simulink model "const_vel_static_obst"  (R2023b)
settings: Solver=ode4  StartTime=0.0  StopTime=50  FixedStep=1e-3  RelTol=1e-3  EnableMultiTasking=on
values from neighbouring files (symbols this model uses):
  Ts = 0.01    [const_vel_static_obst_run.m]    (also in const_vel_wall_run.m; run_acceleration.m; run_template.m; simple_const_vel_run.m)
  V_ref = 50/3.6    (= 13.8888888889)    [const_vel_static_obst_run.m]    (also in const_vel_wall_run.m; run_acceleration.m = 27.7777777778; run_template.m = 27.7777777778; simple_const_vel_run.m)
  X0 = [V_ref 0 0 0 0 0 0]    [const_vel_static_obst_run.m]    (also in const_vel_wall_run.m; run_acceleration.m = [V_ref 0 0 0 0 0]; run_template.m; simple_const_vel_run.m)
undefined symbols (not defined in the file or in its folder): data, init, input
settings Model: Creator=bshyrokau  LastModifiedBy=maart
settings SolverCC: AlgebraicLoopSolver=TrustRegion  AutoInsertRateTranBlk=on
settings DataIOCC: SaveOutput=off  SignalLogging=off  DSMLogging=off  SaveTime=off  ReturnWorkspaceOutputs=off
settings OptimizationCC: ReuseModelBlockBuffer=off  LifeSpan=inf
settings DebuggingCC: UnconnectedInputMsg=warning  UnconnectedOutputMsg=warning  UnconnectedLineMsg=warning  AllowSymbolicDim=off  SFUnexpectedBacktrackingDiag=warning  SFNoUnconditionalDefaultTransitionDiag=warning  SFExecutionAtInitializationDiag=none  ArithmeticOperatorsInVariantConditions=warning
settings ModelReferenceCC: EnableRefExpFcnMdlSchedulingChecks=on  PropagateSignalLabelsOutOfModel=off
settings SFSimCC: SimUseLocalCustomCode=off  CustomCodeUndefinedFunction=UseInterfaceOnly
settings RTWCC: RTWUseLocalCustomCode=off
settings CodeAppCC: StateflowObjectComments=on
settings GRTTargetCC: TargetLangStandard=C89/C90 (ANSI)
settings ConfigComp: CovMetricSettings=dw  CovSaveCumulativeToWorkspaceVar=on  CovSaveSingleToWorkspaceVar=on  CovExternalEMLEnable=off
settings SimscapeCC: SimscapeNormalizeSystem=off
settings ConfigurationSet: Description=SimMechanics 2G

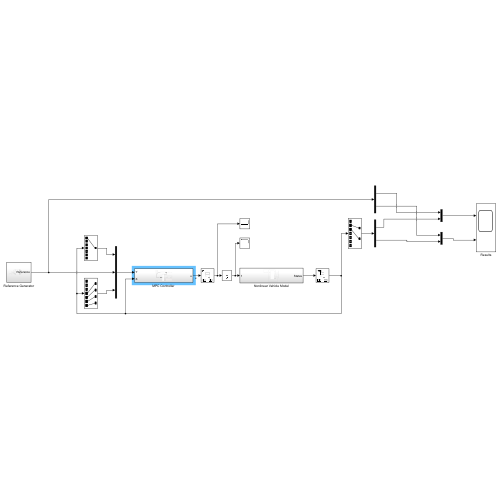
[thumbnail: Simulink's stored preview of the top-level diagram]
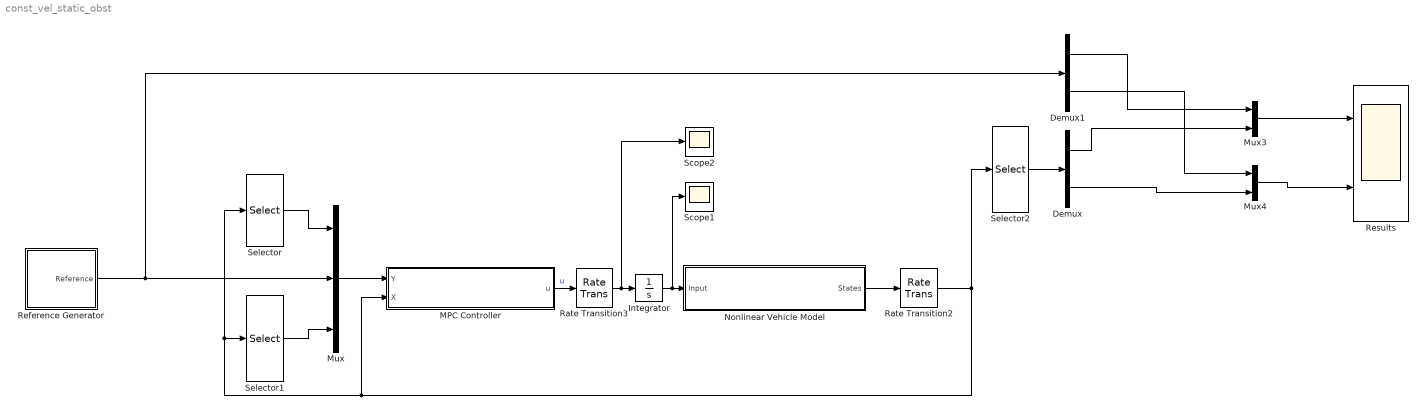
== system const_vel_static_obst ==
  Demux : Demux  Outputs=2
  Demux1 : Demux  Outputs=2
  Integrator : Integrator
  "MPC Controller " : Subsystem
  Mux : Mux  Inputs=3
  Mux3 : Mux  Inputs=2
  Mux4 : Mux  Inputs=2
  Nonlinear Vehicle Model : Subsystem
  Rate Transition2 : RateTransition  InitialCondition=X0  OutPortSampleTime=Ts
  Rate Transition3 : RateTransition  InitialCondition=[0]
  Reference Generator : Subsystem
  Results : Scope  NumInputPorts=2
  Scope1 : Scope
  Scope2 : Scope
  Selector : Selector  InputPortWidth=7  IndexOptions=Index vector (dialog)  Indices=[1]  OutputSizes=1
  Selector1 : Selector  InputPortWidth=7  IndexOptions=Index vector (dialog)  Indices=[4,5,6,7]  OutputSizes=1
  Selector2 : Selector  InputPortWidth=7  IndexOptions=Index vector (dialog)  Indices=[2,3]  OutputSizes=1
  wires:
  Nonlinear Vehicle Model/1(States) -> Rate Transition2/1
  Rate Transition2/1 -> "MPC Controller "/2(X), Selector/1, Selector1/1, Selector2/1
  "MPC Controller "/1(u) -> Rate Transition3/1  "u"
  Mux/1 -> "MPC Controller "/1(Y)
  Selector1/1 -> Mux/3
  Selector2/1 -> Demux/1
  Demux1/1 -> Mux3/1
  Demux1/2 -> Mux4/1
  Demux/1 -> Mux3/2
  Demux/2 -> Mux4/2
  Reference Generator/1(Reference) -> Demux1/1, Mux/2
  Selector/1 -> Mux/1
  Rate Transition3/1 -> Scope2/1, Integrator/1
  Integrator/1 -> Scope1/1, Nonlinear Vehicle Model/1(Input)
  Mux3/1 -> Results/1
  Mux4/1 -> Results/2

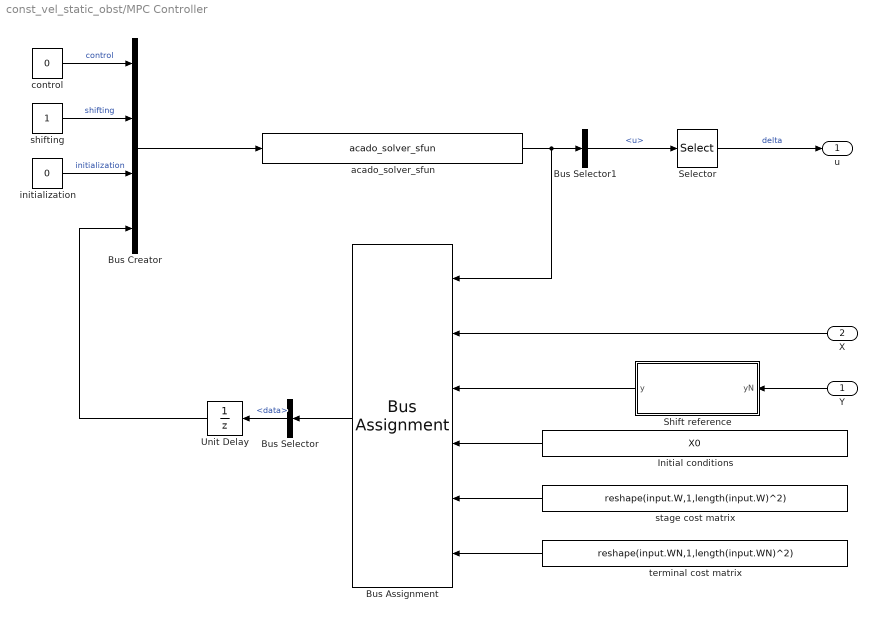
== system const_vel_static_obst/MPC Controller  ==
  Y : Inport
  X : Inport  Port=2
  Bus Assignment : BusAssignment  AssignedSignals=data.x0,data.y,data.yN,data.W,data.WN
  Bus Creator : BusCreator  Inputs=4  OutDataTypeStr=Bus: ACADOinput
  Bus Selector : BusSelector  OutputSignals=data
  Bus Selector1 : BusSelector  OutputSignals=data.u
  Initial conditions : Constant  Value=X0
  Selector : Selector  InputPortWidth=Np  IndexOptions=Starting index (dialog)  Indices=1  OutputSizes=1
  Shift reference : MATLAB Function  TreatAsAtomicUnit=on
  Unit Delay : UnitDelay  InitialCondition=init  SampleTime=Ts  HasFrameUpgradeWarning=on
  acado_solver_sfun : S-Function  FunctionName=acado_solver_sfun  SFunctionDeploymentMode=off  EnableBusSupport=off  mask(Legacy Function){SFunctionSpec=acado_step(ACADOinput u1[1], ACADOoutput y1[1]), ShowSpec=on}
      mask prompts: ShowSpec "Display function specification"
      mask help:
      | This block allows you to call the legacy functions specified by the following Legacy Code Tool definition:
      | def.SFunctionName = 'acado_solver_sfun';
      | def.OutputFcnSpec = 'acado_step(ACADOinput u1[1], ACADOoutput y1[1])';
      | def.StartFcnSpec = 'acado_initialize( void )';
      | def.TerminateFcnSpec = 'acado_cleanup( void )';
      | def.HeaderFiles = {'acado_common.h', 'acado_solver_sfunction.h'};
      | def.SourceFiles = {'acado_solver.c', 'acado_integrator.c', 'acado_auxiliary_functions.c', 'acado_solver_sfunction.c', 'acado_qpoases3_interface.c', 'qpoases3\src\Bounds.c', 'qpoases3\src\Constraints.c', 'qpoases3\src\Indexlist.c', 'qpoases3\src\Matrices.c', 'qpoases3\src\MessageHandling.c', 'qpoases3\src\Options.c', 'qpoases3\src\Flipper.c', 'qpoases3\src\QProblem.c', 'qpoases3\src\QProblemB.c', 'qpoases3\src\Utils.c'};
      mask Help: <p>This block was generated automatically by the Legacy Code Tool. For detailed help on this tool, call<a href="matlab:legacy_code('help')"> legacy_code('help')</a>.</p>
      mask Callback ShowSpec:
      | if strcmp(get_param(gcbh, 'ShowSpec'), 'on')
      |   set_param(gcbh, 'MaskDisplay', sprintf('fprintf(''%s'');', get_param(gcbh, 'SFunctionSpec')));
      | else
      |   set_param(gcbh, 'MaskDisplay', sprintf('fprintf(''%s'');', get_param(gcbh, 'FunctionName')));
      | end
      mask Display: fprintf('acado_step(ACADOinput u1[1], ACADOoutput y1[1])');
  control : Constant  Value=0  OutDataTypeStr=int32
  initialization : Constant  Value=0  OutDataTypeStr=int32
  shifting : Constant  OutDataTypeStr=int32
  stage cost matrix : Constant  Value=reshape(input.W,1,length(input.W)^2)
  terminal cost matrix : Constant  Value=reshape(input.WN,1,length(input.WN)^2)
  u : Outport
  wires:
  control/1 -> Bus Creator/1  "control"
  Bus Selector1/1 -> Selector/1  "<u>"
  initialization/1 -> Bus Creator/3  "initialization"
  acado_solver_sfun/1 -> Bus Selector1/1, Bus Assignment/1
  shifting/1 -> Bus Creator/2  "shifting"
  X/1 -> Bus Assignment/2
  Bus Assignment/1 -> Bus Selector/1
  terminal cost matrix/1 -> Bus Assignment/6
  Initial conditions/1 -> Bus Assignment/4
  Shift reference/1(y) -> Bus Assignment/3
  stage cost matrix/1 -> Bus Assignment/5
  Bus Selector/1 -> Unit Delay/1  "<data>"
  Unit Delay/1 -> Bus Creator/4
  Bus Creator/1 -> acado_solver_sfun/1
  Selector/1 -> u/1  "delta"
  Y/1 -> Shift reference/1(yN)

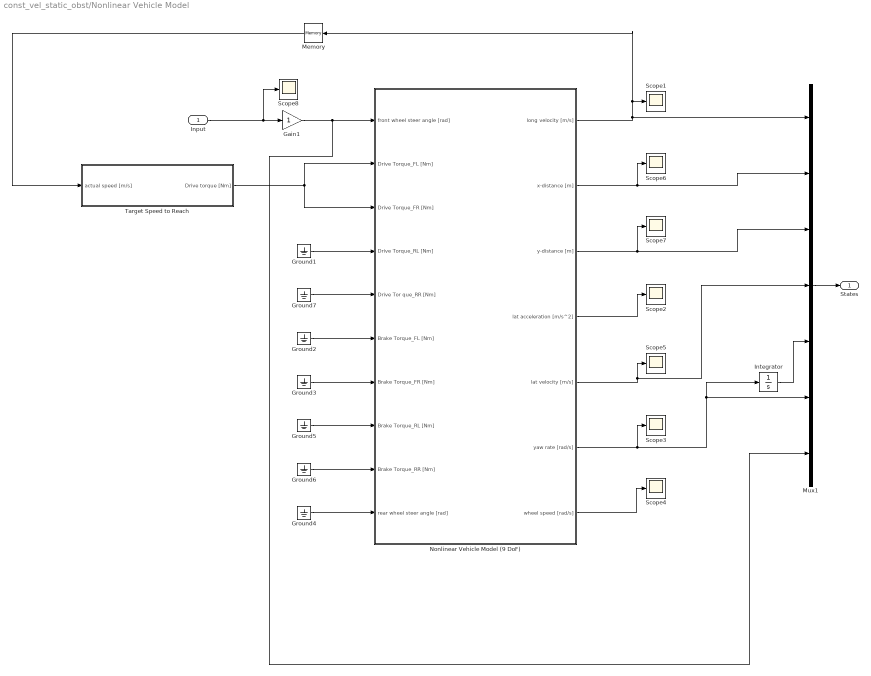
== system const_vel_static_obst/Nonlinear Vehicle Model ==
  Input : Inport
  Gain1 : Gain
  Ground{1..7} (7 alike) : Ground
  Integrator : Integrator
  Memory : Memory
  Mux1 : Mux  Inputs=7
  Nonlinear Vehicle Model (9 DoF) : Subsystem
      mask help: Simulink:masks:GenSFuncDesc_MD
      mask Help: eval('feval(''rtwprivate'',''rtwhelpview'',''rtw_sfcn_block'')');
  Scope{1..8} (8 alike) : Scope
  Target Speed to Reach : Subsystem
  States : Outport
  wires:
  Nonlinear Vehicle Model (9 DoF)/2(x-distance [m]) -> Mux1/2, Scope6/1
  Input/1 -> Scope8/1, Gain1/1
  Nonlinear Vehicle Model (9 DoF)/5(lat velocity [m/s]) -> Scope5/1, Mux1/4
  Ground3/1 -> Nonlinear Vehicle Model (9 DoF)/7(Brake Torque_FR [Nm])
  Nonlinear Vehicle Model (9 DoF)/3(y-distance [m]) -> Mux1/3, Scope7/1
  Nonlinear Vehicle Model (9 DoF)/1(long velocity [m/s]) -> Memory/1, Scope1/1, Mux1/1
  Nonlinear Vehicle Model (9 DoF)/4(lat acceleration [m/s^2]) -> Scope2/1
  Nonlinear Vehicle Model (9 DoF)/6(yaw rate [rad/s]) -> Scope3/1, Mux1/6, Integrator/1
  Ground2/1 -> Nonlinear Vehicle Model (9 DoF)/6(Brake Torque_FL [Nm])
  Mux1/1 -> States/1
  Integrator/1 -> Mux1/5
  Ground4/1 -> Nonlinear Vehicle Model (9 DoF)/10(rear wheel steer angle [rad])
  Ground5/1 -> Nonlinear Vehicle Model (9 DoF)/8(Brake Torque_RL [Nm])
  Ground6/1 -> Nonlinear Vehicle Model (9 DoF)/9(Brake Torque_RR [Nm])
  Nonlinear Vehicle Model (9 DoF)/7(wheel speed [rad/s]) -> Scope4/1
  Target Speed to Reach/1(Drive torque [Nm]) -> Nonlinear Vehicle Model (9 DoF)/3(Drive Torque_FR [Nm]), Nonlinear Vehicle Model (9 DoF)/2(Drive Torque_FL [Nm])
  Gain1/1 -> Nonlinear Vehicle Model (9 DoF)/1(front wheel steer angle [rad]), Mux1/7
  Ground7/1 -> Nonlinear Vehicle Model (9 DoF)/5(Drive Tor	que_RR [Nm])
  Ground1/1 -> Nonlinear Vehicle Model (9 DoF)/4(Drive Torque_RL [Nm])
  Memory/1 -> Target Speed to Reach/1(actual speed [m/s])

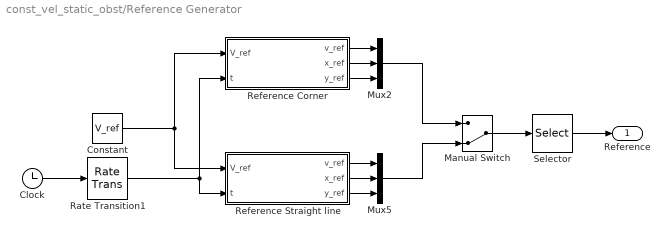
== system const_vel_static_obst/Reference Generator ==
  Clock : Clock
  Constant : Constant  Value=V_ref
  Manual Switch : ManualSwitch  CurrentSetting=0
  Mux2 : Mux  Inputs=3
  Mux5 : Mux  Inputs=3
  Rate Transition1 : RateTransition  OutPortSampleTime=Ts
  Reference Corner : MATLAB Function  TreatAsAtomicUnit=on
  Reference Straight line : MATLAB Function  TreatAsAtomicUnit=on
  Selector : Selector  InputPortWidth=3  IndexOptions=Index vector (dialog)  Indices=[2 3]  OutputSizes=1
  Reference : Outport
  wires:
  Clock/1 -> Rate Transition1/1
  Reference Corner/2(x_ref) -> Mux2/2
  Reference Corner/1(v_ref) -> Mux2/1
  Rate Transition1/1 -> Reference Straight line/2(t), Reference Corner/2(t)
  Constant/1 -> Reference Straight line/1(V_ref), Reference Corner/1(V_ref)
  Reference Corner/3(y_ref) -> Mux2/3
  Reference Straight line/1(v_ref) -> Mux5/1
  Reference Straight line/2(x_ref) -> Mux5/2
  Reference Straight line/3(y_ref) -> Mux5/3
  Selector/1 -> Reference/1
  Mux5/1 -> Manual Switch/2
  Mux2/1 -> Manual Switch/1
  Manual Switch/1 -> Selector/1

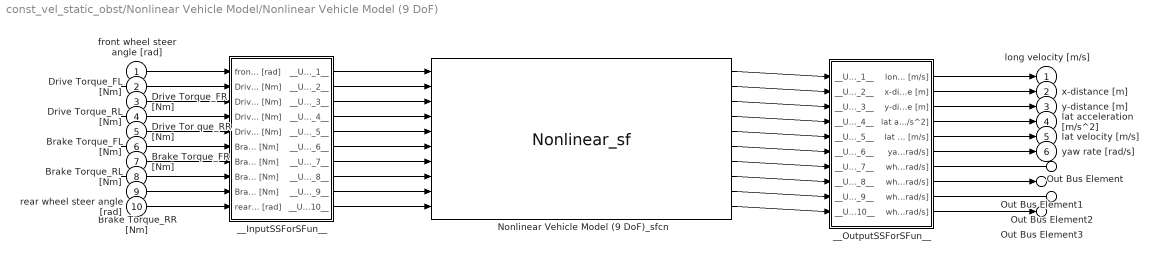
== system const_vel_static_obst/Nonlinear Vehicle Model/Nonlinear Vehicle Model (9 DoF) ==
  front wheel steer angle [rad] : Inport
  Drive Torque_FL [Nm] : Inport  Port=2
  Drive Torque_FR [Nm] : Inport  Port=3
  Drive Torque_RL [Nm] : Inport  Port=4
  Drive Tor	que_RR [Nm] : Inport  Port=5
  Brake Torque_FL [Nm] : Inport  Port=6
  Brake Torque_FR [Nm] : Inport  Port=7
  Brake Torque_RL [Nm] : Inport  Port=8
  Brake Torque_RR [Nm] : Inport  Port=9
  rear wheel steer angle [rad] : Inport  Port=10
  Nonlinear Vehicle Model (9 DoF)_sfcn : S-Function  FunctionName=Nonlinear_sf  SFunctionModules=""  SFunctionDeploymentMode=off  EnableBusSupport=off  mask{rtw_sf_name=Nonlinear_sf, showVar=off}
      mask prompts: rtw_sf_name "Simulink:masks:GenSFuncName_MP"; showVar "Simulink:masks:GenSFuncShowModuleList_MP"
      mask help: Simulink:masks:GenSFuncDesc_MD
      mask init:
      | displist = '';
      | if ~strcmp(get_param(gcb, 'FunctionName'), rtw_sf_name);
      |   set_param(gcb, 'FunctionName', rtw_sf_name);
      | end
      | % Check if we are generating code
      | rtw_mode = false;
      | if strcmpi(get_param(bdroot(gcb),'SimulationStatus'),'Initializing')
      | 	rtw_mode = strcmpi(get_param(bdroot(gcb),'BuildingRTWCode'),'on') && ...
      | 		~strcmpi(get_param(bdroot(gcb),'TargetStyle'),'SimulationTarget');
      | end
      | if showVar || rtw_mode
      | 	if exist('rtwsfunc') == 2 | exist('rtwsfunc') == 6
      | 		tmplist = rtwsfunc(rtw_sf_name,gcb);
      | 		tmplist = DAStudio.message('Simulink:masks:GenSFuncListOfModules_IC', tmplist);
      | 	elseif showVar
      | 		tmplist1 = DAStudio.message('Simulink:masks:GenSFuncListOfModules_IC', '');
      |         tmplist2 = DAStudio.message('Simulink:masks:GenSFuncNotLicensed_IC');
      |         tmplist = [tmplist1 tmplist2];
      |  	end
      | end
      | if showVar
      |   displist = tmplist;
      | end
      settings: CopyFcn=|
      | if ~strcmp(get_param(gcb,'Linkstatus'),'none') && ...
      | ~strcmp(get_param(gcb,'Linkstatus'),'implicit')
      |   set_param(gcb,'LinkStatus','none');
      | end
      mask Help: eval('feval(''rtwprivate'',''rtwhelpview'',''rtw_sfcn_block'')');
      mask Display:
      | port_label('input',1,'front wheel steer angle [rad]');
      | port_label('input',2,'Drive Torque_FL [Nm]');
      | port_label('input',3,'Drive Torque_FR [Nm]');
      | port_label('input',4,'Drive Torque_RL [Nm]');
      | port_label('input',5,'Drive Tor	que_RR [Nm]');
      | port_label('input',6,'Brake Torque_FL [Nm]');
      | port_label('input',7,'Brake Torque_FR [Nm]');
      | port_label('input',8,'Brake Torque_RL [Nm]');
      | port_label('input',9,'Brake Torque_RR [Nm]');
      | port_label('input',10,'rear wheel steer angle [rad]');
      | port_label('output',1,'long velocity [m/s]');
      | port_label('output',2,'x-distance [m]');
      | port_label('output',3,'y-distance [m]');
      | port_label('output',4,'lat acceleration [m/s^2]');
      | port_label('output',5,'lat velocity [m/s]');
      | port_label('output',6,'yaw rate [rad/s]');
      | port_label('output',7,'wheel speed FL [rad/s]');
      | port_label('output',8,'wheel speed FR [rad/s]');
      | port_label('output',9,'wheel speed RL [rad/s]');
      | port_label('output',10,'wheel speed RR [rad/s]');
  __InputSSForSFun__ : Subsystem
  __OutputSSForSFun__ : Subsystem
  long velocity [m/s] : Outport  VectorParamsAs1DForOutWhenUnconnected=off
  x-distance [m] : Outport  Port=2  VectorParamsAs1DForOutWhenUnconnected=off
  y-distance [m] : Outport  Port=3  VectorParamsAs1DForOutWhenUnconnected=off
  lat acceleration [m/s^2] : Outport  Port=4  VectorParamsAs1DForOutWhenUnconnected=off
  lat velocity [m/s] : Outport  Port=5  VectorParamsAs1DForOutWhenUnconnected=off
  yaw rate [rad/s] : Outport  Port=6  VectorParamsAs1DForOutWhenUnconnected=off
  Out Bus Element : Outport  Port=7  PortName=wheel speed [rad/s]  Element=wheel speed FL [rad/s]
  Out Bus Element1 : Outport  Port=7  PortName=wheel speed [rad/s]  Element=wheel speed FR [rad/s]
  Out Bus Element2 : Outport  Port=7  PortName=wheel speed [rad/s]  Element=wheel speed RL [rad/s]
  Out Bus Element3 : Outport  Port=7  PortName=wheel speed [rad/s]  Element=wheel speed RR [rad/s]
  wires:
  front wheel steer angle [rad]/1 -> __InputSSForSFun__/1(front wheel steer angle [rad])
  Drive Torque_FL [Nm]/1 -> __InputSSForSFun__/2(Drive Torque_FL [Nm])
  Drive Torque_FR [Nm]/1 -> __InputSSForSFun__/3(Drive Torque_FR [Nm])
  Drive Torque_RL [Nm]/1 -> __InputSSForSFun__/4(Drive Torque_RL [Nm])
  Drive Tor	que_RR [Nm]/1 -> __InputSSForSFun__/5(Drive Tor	que_RR [Nm])
  Brake Torque_FL [Nm]/1 -> __InputSSForSFun__/6(Brake Torque_FL [Nm])
  Brake Torque_FR [Nm]/1 -> __InputSSForSFun__/7(Brake Torque_FR [Nm])
  Brake Torque_RL [Nm]/1 -> __InputSSForSFun__/8(Brake Torque_RL [Nm])
  Brake Torque_RR [Nm]/1 -> __InputSSForSFun__/9(Brake Torque_RR [Nm])
  rear wheel steer angle [rad]/1 -> __InputSSForSFun__/10(rear wheel steer angle [rad])
  __InputSSForSFun__/1(__UniqueOutportName__1__) -> Nonlinear Vehicle Model (9 DoF)_sfcn/1
  __InputSSForSFun__/2(__UniqueOutportName__2__) -> Nonlinear Vehicle Model (9 DoF)_sfcn/2
  __InputSSForSFun__/3(__UniqueOutportName__3__) -> Nonlinear Vehicle Model (9 DoF)_sfcn/3
  __InputSSForSFun__/4(__UniqueOutportName__4__) -> Nonlinear Vehicle Model (9 DoF)_sfcn/4
  __InputSSForSFun__/5(__UniqueOutportName__5__) -> Nonlinear Vehicle Model (9 DoF)_sfcn/5
  __InputSSForSFun__/6(__UniqueOutportName__6__) -> Nonlinear Vehicle Model (9 DoF)_sfcn/6
  __InputSSForSFun__/7(__UniqueOutportName__7__) -> Nonlinear Vehicle Model (9 DoF)_sfcn/7
  __InputSSForSFun__/8(__UniqueOutportName__8__) -> Nonlinear Vehicle Model (9 DoF)_sfcn/8
  __InputSSForSFun__/9(__UniqueOutportName__9__) -> Nonlinear Vehicle Model (9 DoF)_sfcn/9
  __InputSSForSFun__/10(__UniqueOutportName__10__) -> Nonlinear Vehicle Model (9 DoF)_sfcn/10
  Nonlinear Vehicle Model (9 DoF)_sfcn/1 -> __OutputSSForSFun__/1(__UniqueInportName__1__)
  Nonlinear Vehicle Model (9 DoF)_sfcn/2 -> __OutputSSForSFun__/2(__UniqueInportName__2__)
  Nonlinear Vehicle Model (9 DoF)_sfcn/3 -> __OutputSSForSFun__/3(__UniqueInportName__3__)
  Nonlinear Vehicle Model (9 DoF)_sfcn/4 -> __OutputSSForSFun__/4(__UniqueInportName__4__)
  Nonlinear Vehicle Model (9 DoF)_sfcn/5 -> __OutputSSForSFun__/5(__UniqueInportName__5__)
  Nonlinear Vehicle Model (9 DoF)_sfcn/6 -> __OutputSSForSFun__/6(__UniqueInportName__6__)
  Nonlinear Vehicle Model (9 DoF)_sfcn/7 -> __OutputSSForSFun__/7(__UniqueInportName__7__)
  Nonlinear Vehicle Model (9 DoF)_sfcn/8 -> __OutputSSForSFun__/8(__UniqueInportName__8__)
  Nonlinear Vehicle Model (9 DoF)_sfcn/9 -> __OutputSSForSFun__/9(__UniqueInportName__9__)
  Nonlinear Vehicle Model (9 DoF)_sfcn/10 -> __OutputSSForSFun__/10(__UniqueInportName__10__)
  __OutputSSForSFun__/1(long velocity [m/s]) -> long velocity [m/s]/1
  __OutputSSForSFun__/2(x-distance [m]) -> x-distance [m]/1
  __OutputSSForSFun__/3(y-distance [m]) -> y-distance [m]/1
  __OutputSSForSFun__/4(lat acceleration [m/s^2]) -> lat acceleration [m/s^2]/1
  __OutputSSForSFun__/5(lat velocity [m/s]) -> lat velocity [m/s]/1
  __OutputSSForSFun__/6(yaw rate [rad/s]) -> yaw rate [rad/s]/1
  __OutputSSForSFun__/7(wheel speed FL [rad/s]) -> Out Bus Element/1
  __OutputSSForSFun__/8(wheel speed FR [rad/s]) -> Out Bus Element1/1
  __OutputSSForSFun__/9(wheel speed RL [rad/s]) -> Out Bus Element2/1
  __OutputSSForSFun__/10(wheel speed RR [rad/s]) -> Out Bus Element3/1

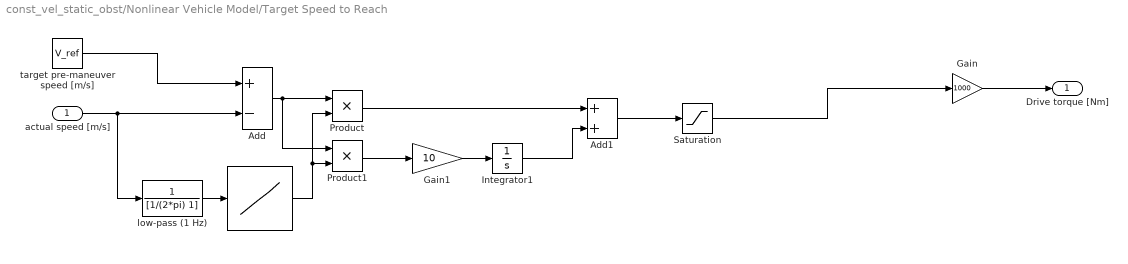
== system const_vel_static_obst/Nonlinear Vehicle Model/Target Speed to Reach ==
  actual speed [m/s] : Inport
  " " : Lookup_n-D  NumberOfTableDimensions=1  BreakpointsForDimension1="[-10  0  10 30]"  IndexSearchMethod=Linear search  Table=[0.1 0.1 1 1]  ExtrapMethod=Clip  RemoveProtectionInput=on  UseLastTableValue=on  RndMeth=Simplest
  Add : Sum  Inputs=+-
  Add1 : Sum
  Gain : Gain  Gain=1000
  Gain1 : Gain  Gain=10
  Integrator1 : Integrator  LimitOutput=on  UpperSaturationLimit=0.1  LowerSaturationLimit=-0.1
  Product : Product  RndMeth=Zero
  Product1 : Product  RndMeth=Zero
  Saturation : Saturate  UpperLimit=1  LowerLimit=0
  low-pass (1 Hz) : TransferFcn  Denominator=[1/(2*pi) 1]
  "target pre-maneuver speed [m/s] " : Constant  Value=V_ref
  Drive torque [Nm] : Outport
  wires:
  actual speed [m/s]/1 -> low-pass (1 Hz)/1, Add/2
  "target pre-maneuver speed [m/s] "/1 -> Add/1
  Gain1/1 -> Integrator1/1
  Product/1 -> Add1/1
  Add/1 -> Product/1, Product1/1
  Product1/1 -> Gain1/1
  " "/1 -> Product1/2, Product/2
  low-pass (1 Hz)/1 -> " "/1
  Add1/1 -> Saturation/1
  Integrator1/1 -> Add1/2
  Saturation/1 -> Gain/1
  Gain/1 -> Drive torque [Nm]/1

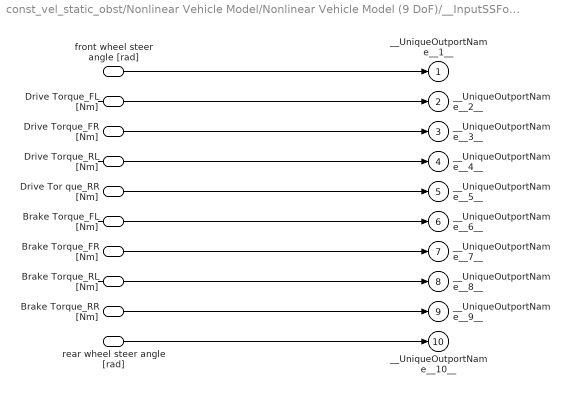
== system const_vel_static_obst/Nonlinear Vehicle Model/Nonlinear Vehicle Model (9 DoF)/__InputSSForSFun__ ==
  front wheel steer angle [rad] : Inport
  Drive Torque_FL [Nm] : Inport  Port=2
  Drive Torque_FR [Nm] : Inport  Port=3
  Drive Torque_RL [Nm] : Inport  Port=4
  Drive Tor	que_RR [Nm] : Inport  Port=5
  Brake Torque_FL [Nm] : Inport  Port=6
  Brake Torque_FR [Nm] : Inport  Port=7
  Brake Torque_RL [Nm] : Inport  Port=8
  Brake Torque_RR [Nm] : Inport  Port=9
  rear wheel steer angle [rad] : Inport  Port=10
  __UniqueOutportName__1__ : Outport
  __UniqueOutportName__2__ : Outport  Port=2
  __UniqueOutportName__3__ : Outport  Port=3
  __UniqueOutportName__4__ : Outport  Port=4
  __UniqueOutportName__5__ : Outport  Port=5
  __UniqueOutportName__6__ : Outport  Port=6
  __UniqueOutportName__7__ : Outport  Port=7
  __UniqueOutportName__8__ : Outport  Port=8
  __UniqueOutportName__9__ : Outport  Port=9
  __UniqueOutportName__10__ : Outport  Port=10
  wires:
  front wheel steer angle [rad]/1 -> __UniqueOutportName__1__/1
  Drive Torque_FL [Nm]/1 -> __UniqueOutportName__2__/1
  Drive Torque_FR [Nm]/1 -> __UniqueOutportName__3__/1
  Drive Torque_RL [Nm]/1 -> __UniqueOutportName__4__/1
  Drive Tor	que_RR [Nm]/1 -> __UniqueOutportName__5__/1
  Brake Torque_FL [Nm]/1 -> __UniqueOutportName__6__/1
  Brake Torque_FR [Nm]/1 -> __UniqueOutportName__7__/1
  Brake Torque_RL [Nm]/1 -> __UniqueOutportName__8__/1
  Brake Torque_RR [Nm]/1 -> __UniqueOutportName__9__/1
  rear wheel steer angle [rad]/1 -> __UniqueOutportName__10__/1

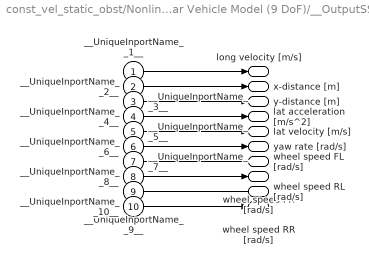
== system const_vel_static_obst/Nonlinear Vehicle Model/Nonlinear Vehicle Model (9 DoF)/__OutputSSForSFun__ ==
  __UniqueInportName__1__ : Inport
  __UniqueInportName__2__ : Inport  Port=2
  __UniqueInportName__3__ : Inport  Port=3
  __UniqueInportName__4__ : Inport  Port=4
  __UniqueInportName__5__ : Inport  Port=5
  __UniqueInportName__6__ : Inport  Port=6
  __UniqueInportName__7__ : Inport  Port=7
  __UniqueInportName__8__ : Inport  Port=8
  __UniqueInportName__9__ : Inport  Port=9
  __UniqueInportName__10__ : Inport  Port=10
  long velocity [m/s] : Outport  VectorParamsAs1DForOutWhenUnconnected=off
  x-distance [m] : Outport  Port=2  VectorParamsAs1DForOutWhenUnconnected=off
  y-distance [m] : Outport  Port=3  VectorParamsAs1DForOutWhenUnconnected=off
  lat acceleration [m/s^2] : Outport  Port=4  VectorParamsAs1DForOutWhenUnconnected=off
  lat velocity [m/s] : Outport  Port=5  VectorParamsAs1DForOutWhenUnconnected=off
  yaw rate [rad/s] : Outport  Port=6  VectorParamsAs1DForOutWhenUnconnected=off
  wheel speed FL [rad/s] : Outport  Port=7  VectorParamsAs1DForOutWhenUnconnected=off
  wheel speed FR [rad/s] : Outport  Port=8  VectorParamsAs1DForOutWhenUnconnected=off
  wheel speed RL [rad/s] : Outport  Port=9  VectorParamsAs1DForOutWhenUnconnected=off
  wheel speed RR [rad/s] : Outport  Port=10  VectorParamsAs1DForOutWhenUnconnected=off
  wires:
  __UniqueInportName__1__/1 -> long velocity [m/s]/1
  __UniqueInportName__2__/1 -> x-distance [m]/1
  __UniqueInportName__3__/1 -> y-distance [m]/1
  __UniqueInportName__4__/1 -> lat acceleration [m/s^2]/1
  __UniqueInportName__5__/1 -> lat velocity [m/s]/1
  __UniqueInportName__6__/1 -> yaw rate [rad/s]/1
  __UniqueInportName__7__/1 -> wheel speed FL [rad/s]/1
  __UniqueInportName__8__/1 -> wheel speed FR [rad/s]/1
  __UniqueInportName__9__/1 -> wheel speed RL [rad/s]/1
  __UniqueInportName__10__/1 -> wheel speed RR [rad/s]/1

== matlab function const_vel_static_obst/Reference Generator/Reference Corner ==
  data: V_ref input; v_ref output; x_ref output; y_ref output; t input
function [v_ref, x_ref, y_ref] = reference(V_ref,t)
%#codegen
% Reference Real-Time Function
% Inputs:
%   V_ref - Reference speed in m/s
%   t     - Current simulation time in seconds
% Outputs:
%   v_ref - Reference speed in m/s
%   x_ref - Reference x position in meters
%   y_ref - Reference y position in meters

    % Call the external reference function
    [v_ref, x_ref, y_ref] = reference_corner(V_ref,t);
end

== matlab function const_vel_static_obst/MPC Controller /Shift reference ==
  data: y output; yN input; Np parameter
function y = shift_reference(yN,Np)

y=repmat([yN;0],Np,1)';

end

== matlab function const_vel_static_obst/Reference Generator/Reference Straight line ==
  data: V_ref input; v_ref output; x_ref output; y_ref output; t input
function [v_ref, x_ref, y_ref] = reference(V_ref,t)
%#codegen
% Reference Real-Time Function
% Inputs:
%   V_ref - Reference speed in m/s
%   t     - Current simulation time in seconds
% Outputs:
%   v_ref - Reference speed in m/s
%   x_ref - Reference x position in meters
%   y_ref - Reference y position in meters

    % Call the external reference function
    [v_ref, x_ref, y_ref] = reference_real_time(V_ref,t);
end
